simulink model "TurnLightArb"  (R2020b)
settings: Solver=FixedStepDiscrete  StartTime=0.0  StopTime=10.0  FixedStep=0.01  RelTol=1e-3
settings Model: Creator=Wangjianwen  LastModifiedBy=Wangjianwen
settings DataIOCC: SaveFormat=StructureWithTime
settings OptimizationCC: DefaultParameterBehavior=Inlined  EnhancedBackFolding=on  PassReuseOutputArgsAs=Individual arguments  ZeroExternalMemoryAtStartup=off  ZeroInternalMemoryAtStartup=off  OptimizeBlockOrder=speed  DifferentSizesBufferReuse=on  OptimizationCustomize=off  EfficientTunableParamExpr=on
settings DebuggingCC: ParameterTunabilityLossMsg=error
settings ModelReferenceCC: ModelReferenceNumInstancesAllowed=Single
settings SFSimCC: MATLABDynamicMemAlloc=off
settings RTWCC: Description=AUTOSAR  SystemTargetFile=autosar.tlc  GenCodeOnly=on  TemplateMakefile=ert_default_tmf
settings CodeAppCC: ForceParamTrailComments=on  IgnoreCustomStorageClasses=off  OperatorAnnotations=on  SimulinkDataObjDesc=on  SFDataObjDesc=on  InsertBlockDesc=on
settings STFCustomTargetCC: TargetLangStandard=C99 (ISO)  MultiwordLength=256  GenerateFullHeader=off  ParMdlRefBuildCompliant=on  CompOptLevelCompliant=on  ConcurrentExecutionCompliant=off  IncludeMdlTerminateFcn=off  CombineOutputUpdateFcns=on  SuppressErrorStatus=on  ERTCustomFileBanners=on  SupportNonFinite=off  SupportComplex=off  SupportContinuousTime=off  SupportNonInlinedSFcns=off  RemoveResetFunc=on  ParenthesesLevel=Minimum  MATLABClassNameForMDSCustomization=Simulink.SoftwareTarget.ERTCustomization  CPPClassGenCompliant=off  AutosarCompliant=on  GRTInterface=off  UseToolchainInfoCompliant=on  LookupTableObjectStructAxisOrder=2,1,3,4,...  LUTObjectStructOrderEvenSpacing=Size,Table,Breakpoints  SystemTargetFile=autosar.tlc
settings ERTTargetCC: TargetLangStandard=C99 (ISO)  GenerateFullHeader=off  ConcurrentExecutionCompliant=off  IncludeMdlTerminateFcn=off  SuppressErrorStatus=on  SupportNonFinite=off  SupportComplex=off  ParenthesesLevel=Minimum  ModelStepFunctionPrototypeControlCompliant=off  CPPClassGenCompliant=off  AutosarCompliant=on  LookupTableObjectStructAxisOrder=2,1,3,4,...  LUTObjectStructOrderEvenSpacing=Size,Table,Breakpoints  InlinedParameterPlacement=NonHierarchical  ERTCustomFileTemplate=example_file_process.tlc

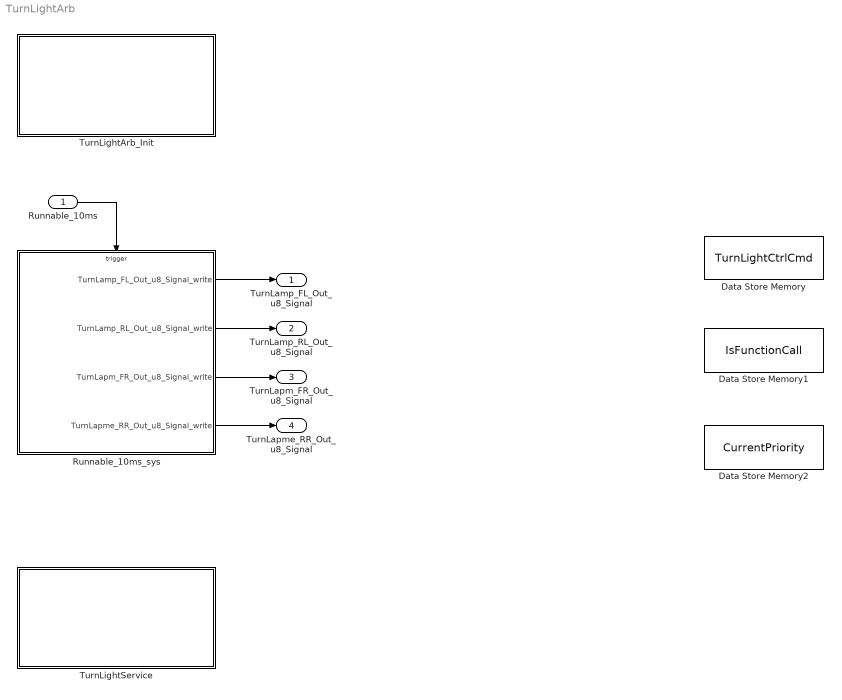
== system TurnLightArb ==
  Runnable_10ms : Inport  SampleTime=0.01  OutputFunctionCall=on
  Data Store Memory : DataStoreMemory  DataStoreName=TurnLightCtrlCmd  ReadBeforeWriteMsg=warning  WriteAfterWriteMsg=warning  WriteAfterReadMsg=warning  ShowAdditionalParam=off  OutDataTypeStr=Bus: TurnLightService
  Data Store Memory1 : DataStoreMemory  DataStoreName=IsFunctionCall  ReadBeforeWriteMsg=warning  WriteAfterWriteMsg=warning  WriteAfterReadMsg=warning  ShowAdditionalParam=off  OutDataTypeStr=boolean
  Data Store Memory2 : DataStoreMemory  DataStoreName=CurrentPriority  ReadBeforeWriteMsg=warning  WriteAfterWriteMsg=warning  WriteAfterReadMsg=warning  ShowAdditionalParam=off  OutDataTypeStr=uint8
  Runnable_10ms_sys : Subsystem
  TurnLightArb_Init : Subsystem
  TurnLightService : Subsystem
  TurnLamp_FL_Out_u8_Signal : Outport  OutDataTypeStr=uint8  PortDimensions=1
  TurnLamp_RL_Out_u8_Signal : Outport  Port=2  OutDataTypeStr=uint8  PortDimensions=1
  TurnLapm_FR_Out_u8_Signal : Outport  Port=3  OutDataTypeStr=uint8  PortDimensions=1
  TurnLapme_RR_Out_u8_Signal : Outport  Port=4  OutDataTypeStr=uint8  PortDimensions=1
  wires:
  Runnable_10ms_sys/1(TurnLamp_FL_Out_u8_Signal_write) -> TurnLamp_FL_Out_u8_Signal/1
  Runnable_10ms_sys/2(TurnLamp_RL_Out_u8_Signal_write) -> TurnLamp_RL_Out_u8_Signal/1
  Runnable_10ms_sys/3(TurnLapm_FR_Out_u8_Signal_write) -> TurnLapm_FR_Out_u8_Signal/1
  Runnable_10ms_sys/4(TurnLapme_RR_Out_u8_Signal_write) -> TurnLapme_RR_Out_u8_Signal/1
  Runnable_10ms/1 -> Runnable_10ms_sys/Trigger

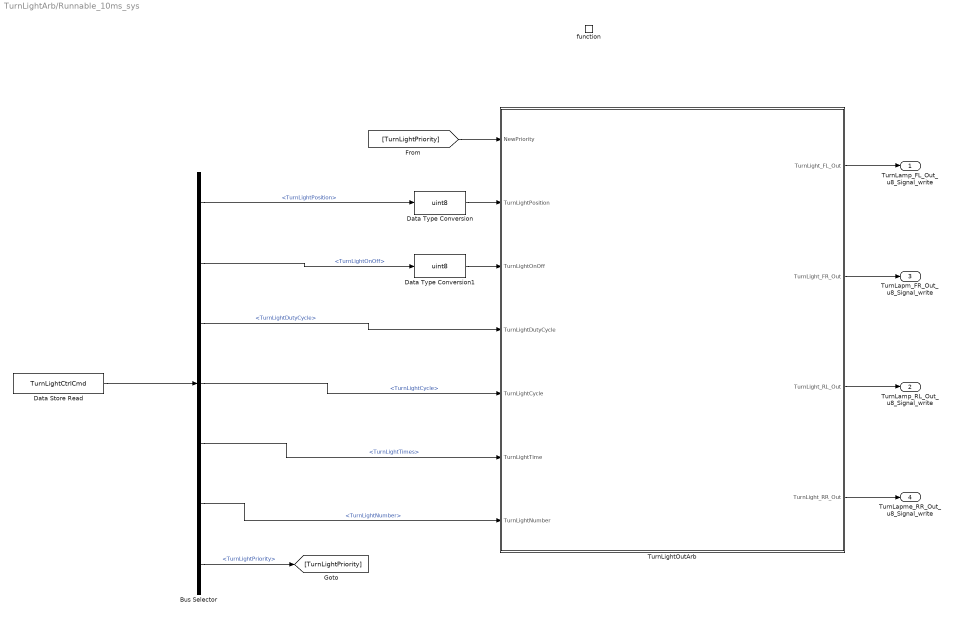
== system TurnLightArb/Runnable_10ms_sys ==
  function : TriggerPort  TriggerType=function-call  VariantControl=(inherit)  SampleTimeType=periodic  SampleTime=-1
  Bus Selector : BusSelector  OutputSignals=TurnLightPosition,TurnLightOnOff,TurnLightDutyCycle,TurnLightCycle,TurnLightTimes,TurnLightNumber,TurnLightPriority
  Data Store Read : DataStoreRead  DataStoreName=TurnLightCtrlCmd
  Data Type Conversion : DataTypeConversion  OutDataTypeStr=uint8
  Data Type Conversion1 : DataTypeConversion  OutDataTypeStr=uint8
  TurnLightOutArb : Stateflow chart  TreatAsAtomicUnit=on
  TurnLamp_FL_Out_u8_Signal_write : Outport
      settings: EnsureOutportIsVirtual=on
  TurnLamp_RL_Out_u8_Signal_write : Outport  Port=2
      settings: EnsureOutportIsVirtual=on
  TurnLapm_FR_Out_u8_Signal_write : Outport  Port=3
      settings: EnsureOutportIsVirtual=on
  TurnLapme_RR_Out_u8_Signal_write : Outport  Port=4
      settings: EnsureOutportIsVirtual=on
  wires:
  TurnLightOutArb/1(TurnLight_FL_Out) -> TurnLamp_FL_Out_u8_Signal_write/1
  TurnLightOutArb/3(TurnLight_RL_Out) -> TurnLamp_RL_Out_u8_Signal_write/1
  TurnLightOutArb/2(TurnLight_FR_Out) -> TurnLapm_FR_Out_u8_Signal_write/1
  TurnLightOutArb/4(TurnLight_RR_Out) -> TurnLapme_RR_Out_u8_Signal_write/1
  Data Store Read/1 -> Bus Selector/1
  Bus Selector/7 -> [TurnLightPriority]  "<TurnLightPriority>"
  [TurnLightPriority] -> TurnLightOutArb/1(NewPriority)
  Bus Selector/3 -> TurnLightOutArb/4(TurnLightDutyCycle)  "<TurnLightDutyCycle>"
  Bus Selector/4 -> TurnLightOutArb/5(TurnLightCycle)  "<TurnLightCycle>"
  Bus Selector/5 -> TurnLightOutArb/6(TurnLightTime)  "<TurnLightTimes>"
  Bus Selector/6 -> TurnLightOutArb/7(TurnLightNumber)  "<TurnLightNumber>"
  Bus Selector/1 -> Data Type Conversion/1  "<TurnLightPosition>"
  Data Type Conversion/1 -> TurnLightOutArb/2(TurnLightPosition)
  Bus Selector/2 -> Data Type Conversion1/1  "<TurnLightOnOff>"
  Data Type Conversion1/1 -> TurnLightOutArb/3(TurnLightOnOff)

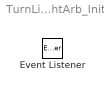
== system TurnLightArb/TurnLightArb_Init ==
  Event Listener : EventListener  EventName=reset

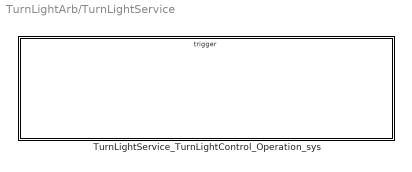
== system TurnLightArb/TurnLightService ==
  TurnLightService_TurnLightControl_Operation_sys : Subsystem

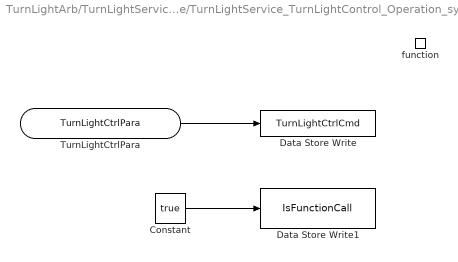
== system TurnLightArb/TurnLightService/TurnLightService_TurnLightControl_Operation_sys ==
  function : TriggerPort  TriggerType=function-call  IsSimulinkFunction=on  FunctionName=TurnLightService_TurnLightControl_Operation  VariantControl=(inherit)
  Constant : Constant  Value=true  OutDataTypeStr=boolean
  Data Store Write : DataStoreWrite  DataStoreName=TurnLightCtrlCmd
  Data Store Write1 : DataStoreWrite  DataStoreName=IsFunctionCall
  TurnLightCtrlPara : ArgIn  OutDataTypeStr=Bus: TurnLightService  ArgumentName=TurnLightCtrlPara
  wires:
  TurnLightCtrlPara/1 -> Data Store Write/1
  Constant/1 -> Data Store Write1/1

== stateflow chart TurnLightArb/Runnable_10ms_sys/TurnLightOutArb ==
  state CheckPriority
    en:
    CheckPriority_flow();
  state JurgeOutputMode [function]
    (default) -> (junction 330)
    (junction 330) -> (junction 332) : { aVarTruthTableCondition_1 = (TurnLightPosition ==ComplexTurnLightPositionType.LEFT); }
    (junction 332) -> (junction 334) : { aVarTruthTableCondition_2 = (TurnLightPosition ==ComplexTurnLightPositionType.RIGHT); }
    (junction 334) -> (junction 336) : { aVarTruthTableCondition_3 = (TurnLightPosition ==ComplexTurnLightPositionType.ALL); }
    (junction 336) -> (junction 338) : { aVarTruthTableCondition_4 = (TurnLightPosition ==ComplexTurnLightPositionType.FRONT_LEFT); }
    (junction 338) -> (junction 340) : { aVarTruthTableCondition_5 = (TurnLightPosition ==ComplexTurnLightPositionType.FRONT_RIGHT); }
    (junction 340) -> (junction 342) : { aVarTruthTableCondition_6 = (TurnLightPosition ==ComplexTurnLightPositionType.REAR_LEFT); }
    (junction 342) -> (junction 344) : { aVarTruthTableCondition_7 = (TurnLightPosition ==ComplexTurnLightPositionType.REAR_RIGHT); }
    (junction 344) -> (junction 346) : { aVarTruthTableCondition_8 = (TurnLightOnOff==ComplexTurnLightONOFFType.OFF); }
    (junction 346) -> (junction 348) : { aVarTruthTableCondition_9 = (TurnLightOnOff==ComplexTurnLightONOFFType.ON); }
    (junction 348) -> (junction 350) : { aVarTruthTableCondition_10 = (TurnLightDutyCycle ==0); }
    (junction 350) -> (junction 352) : { aVarTruthTableCondition_11 = (TurnLightCycle==8); }
    (junction 352) -> (junction 354) : { aVarTruthTableCondition_12 = (TurnLightCycle==4); }
    (junction 354) -> (junction 356) : { aVarTruthTableCondition_13 = (TurnLightTime ==0); }
    (junction 356) -> (junction 358) : { aVarTruthTableCondition_14 = (TurnLightNumber==0); }
    (junction 358) -> (junction 360) : { aVarTruthTableCondition_15 = (TurnLightNumber==3); }
    (junction 360) -> (junction 362) [order 1] : [aVarTruthTableCondition_3 && aVarTruthTableCondition_8]
    (junction 362) -> (junction 364) : {
        | /* 'ALL_OFF': */
        | TurnLight_FL_Out = TLOUT_OFF;TurnLight_FR_Out = TLOUT_OFF;TurnLight_RL_Out = TLOUT_OFF;TurnLight_RR_Out = TLOUT_OFF;
        | }
    (junction 360) -> (junction 366) [order 2]
    (junction 366) -> (junction 368) [order 1] : [aVarTruthTableCondition_4 && aVarTruthTableCondition_8]
    (junction 368) -> (junction 370) : {
        | /* 'FL_OFF': */
        | TurnLight_FL_Out  = TLOUT_OFF;
        | }
    (junction 366) -> (junction 372) [order 2]
    (junction 372) -> (junction 374) [order 1] : [aVarTruthTableCondition_5 && aVarTruthTableCondition_8]
    (junction 374) -> (junction 376) : {
        | /* 'FR_OFF': */
        | TurnLight_FR_Out  = TLOUT_OFF;
        | }
    (junction 372) -> (junction 378) [order 2]
    (junction 378) -> (junction 380) [order 1] : [aVarTruthTableCondition_6 && aVarTruthTableCondition_8]
    (junction 380) -> (junction 382) : {
        | /* 'RL_OFF': */
        | TurnLight_RL_Out  = TLOUT_OFF;
        | }
    (junction 378) -> (junction 384) [order 2]
    (junction 384) -> (junction 386) [order 1] : [aVarTruthTableCondition_7 && aVarTruthTableCondition_8]
    (junction 386) -> (junction 388) : {
        | /* 'RR_OFF': */
        | TurnLight_RR_Out   = TLOUT_OFF;
        | }
    (junction 384) -> (junction 390) [order 2]
    (junction 390) -> (junction 392) [order 1] : [aVarTruthTableCondition_1 && aVarTruthTableCondition_9 && aVarTruthTableCondition_10 && aVarTruthTableCondition_11 && !aVarTruthTableCondition_12 && aVarTruthTableCondition_13 && aVarTruthTableCondition_14 && !aVarTruthTableCondition_15]
    (junction 392) -> (junction 394) : {
        | /* 'LEFT_NORMAL_ON': */
        | TurnLight_FL_Out = TLOUT_NORMAL_ON;TurnLight_RL_Out = TLOUT_NORMAL_ON;
        | }
    (junction 390) -> (junction 396) [order 2]
    (junction 396) -> (junction 398) [order 1] : [aVarTruthTableCondition_2 && aVarTruthTableCondition_9 && aVarTruthTableCondition_10 && aVarTruthTableCondition_11 && !aVarTruthTableCondition_12 && aVarTruthTableCondition_13 && aVarTruthTableCondition_14 && !aVarTruthTableCondition_15]
    (junction 398) -> (junction 400) : {
        | /* 'RIGHT_NORMAL_ON': */
        | TurnLight_FR_Out = TLOUT_NORMAL_ON;TurnLight_RR_Out = TLOUT_NORMAL_ON;
        | }
    (junction 396) -> (junction 402) [order 2]
    (junction 402) -> (junction 404) [order 1] : [aVarTruthTableCondition_3 && aVarTruthTableCondition_9 && aVarTruthTableCondition_10 && aVarTruthTableCondition_11 && !aVarTruthTableCondition_12 && aVarTruthTableCondition_13 && aVarTruthTableCondition_14 && !aVarTruthTableCondition_15]
    (junction 404) -> (junction 406) : {
        | /* 'ALL_NORMAL_ON': */
        | TurnLight_FL_Out = TLOUT_NORMAL_ON;TurnLight_RL_Out = TLOUT_NORMAL_ON;
        | TurnLight_FR_Out = TLOUT_NORMAL_ON;TurnLight_RR_Out = TLOUT_NORMAL_ON;
        | }
    (junction 402) -> (junction 408) [order 2]
    (junction 408) -> (junction 410) [order 1] : [aVarTruthTableCondition_1 && aVarTruthTableCondition_9 && aVarTruthTableCondition_10 && aVarTruthTableCondition_11 && !aVarTruthTableCondition_12 && aVarTruthTableCondition_13 && !aVarTruthTableCondition_14 && aVarTruthTableCondition_15]
    (junction 410) -> (junction 412) : {
        | /* 'LEFT_SHORT_ON': */
        | TurnLight_FL_Out = TLOUT_SHORT_ON;TurnLight_RL_Out = TLOUT_SHORT_ON;
        | }
    (junction 408) -> (junction 414) [order 2]
    (junction 414) -> (junction 416) [order 1] : [aVarTruthTableCondition_2 && aVarTruthTableCondition_9 && aVarTruthTableCondition_10 && aVarTruthTableCondition_11 && !aVarTruthTableCondition_12 && aVarTruthTableCondition_13 && !aVarTruthTableCondition_14 && aVarTruthTableCondition_15]
    (junction 416) -> (junction 418) : {
        | /* 'RIGHT_SHORT_ON': */
        | TurnLight_FR_Out = TLOUT_SHORT_ON;TurnLight_RR_Out = TLOUT_SHORT_ON;
        | }
    (junction 414) -> (junction 420) [order 2]
    (junction 420) -> (junction 422) [order 1] : [aVarTruthTableCondition_4 && aVarTruthTableCondition_9 && aVarTruthTableCondition_10 && !aVarTruthTableCondition_11 && aVarTruthTableCondition_12 && aVarTruthTableCondition_13 && aVarTruthTableCondition_14 && !aVarTruthTableCondition_15]
    (junction 422) -> (junction 424) : {
        | /* 'FL_DOUBLE': */
        | TurnLight_FL_Out  = TLOUT_DOUBLE_ON;
        | }
    (junction 420) -> (junction 426) [order 2]
    (junction 426) -> (junction 428) [order 1] : [aVarTruthTableCondition_5 && aVarTruthTableCondition_9 && aVarTruthTableCondition_10 && !aVarTruthTableCondition_11 && aVarTruthTableCondition_12 && aVarTruthTableCondition_13 && aVarTruthTableCondition_14 && !aVarTruthTableCondition_15]
    (junction 428) -> (junction 430) : {
        | /* 'FR_DOUBLE': */
        | TurnLight_FR_Out  = TLOUT_DOUBLE_ON;
        | }
    (junction 426) -> (junction 432) [order 2]
    (junction 432) -> (junction 434) [order 1] : [aVarTruthTableCondition_6 && aVarTruthTableCondition_9 && aVarTruthTableCondition_10 && !aVarTruthTableCondition_11 && aVarTruthTableCondition_12 && aVarTruthTableCondition_13 && aVarTruthTableCondition_14]
    (junction 434) -> (junction 436) : {
        | /* 'RL_DOUBLE': */
        | TurnLight_RL_Out  = TLOUT_DOUBLE_ON;
        | }
    (junction 432) -> (junction 438) [order 2]
    (junction 438) -> (junction 440) : [aVarTruthTableCondition_7 && aVarTruthTableCondition_9 && aVarTruthTableCondition_10 && !aVarTruthTableCondition_11 && aVarTruthTableCondition_12 && aVarTruthTableCondition_13 && aVarTruthTableCondition_14]
    (junction 440) -> (junction 442) : {
        | /* 'RR_DOUBLE': */
        | TurnLight_RR_Out  = TLOUT_DOUBLE_ON;
        | }
  state Idle
  state CheckPriority_flow [function]
    (default) -> (junction 28)
    (junction 28) -> (junction 29) [order 1] : [NewPriority >=CurrentPriority]
    (junction 28) -> (junction 30) [order 2]
    (junction 29) -> (junction 31) : {
        | CurrentPriority = NewPriority;
        | IsFunctionCall = false;
        | JurgeOutputMode();
        | }
    (junction 31) -> (junction 30)
    (junction 30) -> (junction 445)
  (default) -> Idle
  Idle -> CheckPriority : [IsFunctionCall == true]
  CheckPriority -> Idle : [IsFunctionCall == false]
  data: aVarTruthTableCondition_1 temporary boolean =0; aVarTruthTableCondition_2 temporary boolean =0; aVarTruthTableCondition_3 temporary boolean =0; aVarTruthTableCondition_4 temporary boolean =0; aVarTruthTableCondition_5 temporary boolean =0; aVarTruthTableCondition_6 temporary boolean =0; aVarTruthTableCondition_7 temporary boolean =0; aVarTruthTableCondition_8 temporary boolean =0; aVarTruthTableCondition_9 temporary boolean =0; aVarTruthTableCondition_10 temporary boolean =0; aVarTruthTableCondition_11 temporary boolean =0; aVarTruthTableCondition_12 temporary boolean =0; aVarTruthTableCondition_13 temporary boolean =0; aVarTruthTableCondition_14 temporary boolean =0; aVarTruthTableCondition_15 temporary boolean =0; NewPriority input; TurnLightPosition input; TurnLightOnOff input; TurnLightDutyCycle input; TurnLightCycle input; TurnLightTime input; TurnLightNumber input; TurnLight_FL_Out output uint8 size=1 =0; TurnLight_FR_Out output uint8 size=1 =0; TurnLight_RL_Out output uint8 size=1 =0; TurnLight_RR_Out output uint8 size=1 =0; IsFunctionCall data_store_memory; TLOUT_OFF constant uint8 =0; TLOUT_NORMAL_ON constant uint8 =1; TLOUT_DOUBLE_ON constant uint8 =2; TLOUT_SHORT_ON constant uint8 =3; CurrentPriority data_store_memory
